simulink model "dc_motor"  (R2021b)
settings: Solver=VariableStepAuto  StartTime=0.0  StopTime=10.0  RelTol=1e-3
libraries: spsDCVoltageSourceLib x4, spsDCMachineLib x2, spsSeriesRLCBranchLib x2, spspowerguiLib x1
settings Model: Creator=ANKIT  LastModifiedBy=ANKIT

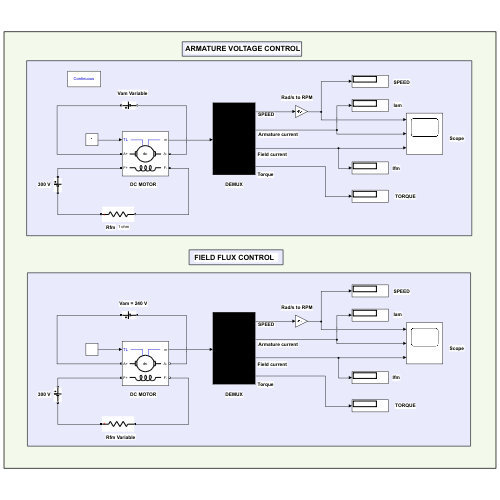
[thumbnail: Simulink's stored preview of the top-level diagram]
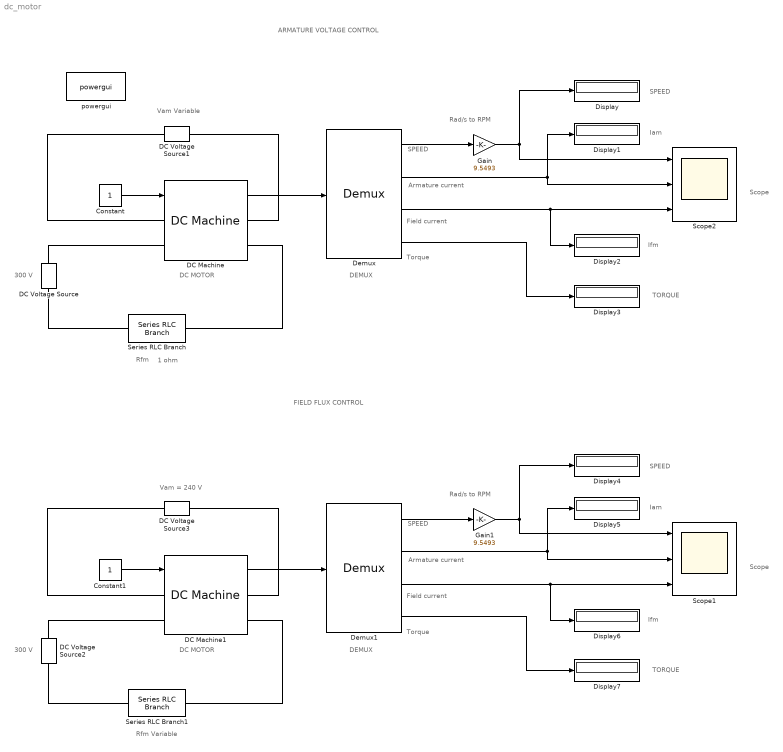
== system dc_motor ==
  note: 1 ohm
  note: Scope
  note: ARMATURE VOLTAGE CONTROL
  note: Rfm Variable
  note: SPEED
  note: 300 V
  note: DC MOTOR
  note: Torque
  note: SPEED
  note: Iam
  note: Rad/s to RPM
  note: Iam
  note: DEMUX
  note: Scope
  note: Ifm
  note: TORQUE
  note: DC MOTOR
  note: Ifm
  note: Field current
  note: Vam = 240 V
  note: Rfm
  note: Field current
  note: TORQUE
  note: Armature current
  note: Armature current
  note: 300 V
  note: Torque
  note: DEMUX
  note: Vam Variable
  note: SPEED
  note: Rad/s to RPM
  note: FIELD FLUX CONTROL
  note: SPEED
  Constant : Constant
  Constant1 : Constant
  DC Machine : spsDCMachineLib/DC Machine  PresetModel=01: 5HP 240V 1750RPM Field:300V  MechanicalLoad=Torque TL  FieldType=Wound  ShowDetailedParameters=on  MeasurementBus=off  RLa=[2.581 0.028]  RLf=[281.2 156]  Laf=0.9483  MachineConstant=Torque constant (N.m/A)  Ke=1.8  Kt=1.8  J=0.02215  Bm=0.002953  Tf=0.5161  w0=1  Ifinit=1.06307583274274  TsPowergui=0  TsBlock=-1
  DC Machine1 : spsDCMachineLib/DC Machine  PresetModel=01: 5HP 240V 1750RPM Field:300V  MechanicalLoad=Torque TL  FieldType=Wound  ShowDetailedParameters=on  MeasurementBus=off  RLa=[2.581 0.028]  RLf=[281.2 156]  Laf=0.9483  MachineConstant=Torque constant (N.m/A)  Ke=1.8  Kt=1.8  J=0.02215  Bm=0.002953  Tf=0.5161  w0=1  Ifinit=1.06307583274274  TsPowergui=0  TsBlock=-1
  DC Voltage Source : spsDCVoltageSourceLib/DC Voltage Source  Amplitude=300  Measurements=None
  DC Voltage Source1 : spsDCVoltageSourceLib/DC Voltage Source  Amplitude=180  Measurements=None
  DC Voltage Source2 : spsDCVoltageSourceLib/DC Voltage Source  Amplitude=300  Measurements=None
  DC Voltage Source3 : spsDCVoltageSourceLib/DC Voltage Source  Amplitude=240  Measurements=None
  Demux : Demux
  Demux1 : Demux
  Display{,1..7} (8 alike) : Display
  Gain : Gain  Gain=9.5493
  Gain1 : Gain  Gain=9.5493
  Scope1 : Scope  NumInputPorts=3
  Scope2 : Scope  NumInputPorts=3
  Series RLC Branch : spsSeriesRLCBranchLib/Series RLC Branch  LConnTagsString=__new0  RConnTagsString=__new0  BranchType=R  Resistance=1  Inductance=1e-3  SetiL0=off  InitialCurrent=0  Capacitance=1e-6  Setx0=off  InitialVoltage=0  Measurements=None
  Series RLC Branch1 : spsSeriesRLCBranchLib/Series RLC Branch  LConnTagsString=__new0  RConnTagsString=__new0  BranchType=R  Resistance=1  Inductance=1e-3  SetiL0=off  InitialCurrent=0  Capacitance=1e-6  Setx0=off  InitialVoltage=0  Measurements=None
  powergui : spspowerguiLib/powergui  Priority=1  SimulationMode=Continuous  SampleTime=50e-6  frequency=60  Iterations=50  frequencyindice=0  Pbase=100e6  ErrMax=1e-4  UnitsV=kV  UnitsW=MW  buscounter=0  FunctionMessages=off  echomessages=off  EnableUseOfTLC=off  CurrentSourceSwitches=off  DisableSnubberDevices=off  DisableRonSwitches=off  DisableVfSwitches=off  DisplayEquations=off  AutomaticDiscreteSolvers=off  SolverType=Tustin/Backward Euler (TBE)  Interpol=off  ExternalGateDelay=off  methode=off  Ts=100  x0status=blocks  SPID=on  SwTol=0  HookPort=off  NonlinearTolerance=1e-4  nMaxIteration=100  ContinueOnMaxIteration=off  RestoreLinks=warning  ResistiveCurrentMeasurement=off  Frange=[0:2:500]  Ylog=off  Xlog=on  ShowGrid=off  save=off  variable=ZData  structure=0  ZoomFFT=off  StartTime=0.0  cycles=1  DisplayStyle=1  fundamental=60  FreqAxis=off  MaxFrequency=1000  frequencyindicesteady=1  RmsSteady=1  display=off
  wires:
  Constant/1 -> DC Machine/1
  Gain1/1 -> Display4/1, Scope1/1
  Demux1/4 -> Display7/1
  Demux1/1 -> Gain1/1
  Constant1/1 -> DC Machine1/1
  DC Machine1/1 -> Demux1/1
  Demux1/2 -> Display5/1, Scope1/2
  DC Machine/1 -> Demux/1
  Demux1/3 -> Display6/1, Scope1/3
  Demux/4 -> Display3/1
  Demux/2 -> Display1/1, Scope2/2
  Demux/3 -> Display2/1, Scope2/3
  Gain/1 -> Display/1, Scope2/1
  Demux/1 -> Gain/1
  connections:
  DC Voltage Source1/RConn1 -- DC Machine/LConn1
  Series RLC Branch/RConn1 -- DC Machine/RConn2
  Series RLC Branch1/RConn1 -- DC Machine1/RConn2
  DC Voltage Source2/LConn1 -- Series RLC Branch1/LConn1
  DC Voltage Source3/LConn1 -- DC Machine1/RConn1
  DC Voltage Source2/RConn1 -- DC Machine1/LConn2
  DC Voltage Source1/LConn1 -- DC Machine/RConn1
  DC Voltage Source3/RConn1 -- DC Machine1/LConn1
  DC Voltage Source/RConn1 -- DC Machine/LConn2
  DC Voltage Source/LConn1 -- Series RLC Branch/LConn1
